simulink subsystem "overwrite_block"  (R2022b)
settings: Solver=VariableStepAuto  StartTime=0.0  StopTime=10.0  RelTol=1e-3
settings Model: Creator=PROSTJP  LastModifiedBy=PROSTJP

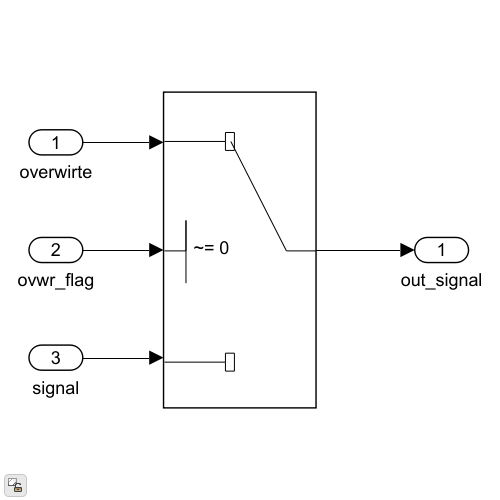
[thumbnail: Simulink's stored preview of the top-level diagram]
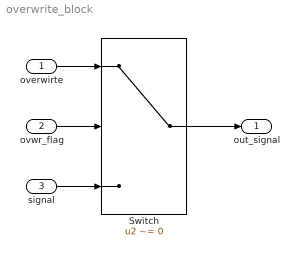
== system overwrite_block ==
  overwirte : Inport
  ovwr_flag : Inport  Port=2
  signal : Inport  Port=3
  Switch : Switch  Criteria=u2 ~= 0  SaturateOnIntegerOverflow=off  InputSameDT=off
  out_signal : Outport
  wires:
  Switch/1 -> out_signal/1
  overwirte/1 -> Switch/1
  ovwr_flag/1 -> Switch/2
  signal/1 -> Switch/3
